simulink model "model_to_linearize"  (R2026a)
settings: Solver=VariableStepAuto
undefined symbols (not defined in the file or in its folder): param
settings Model: Creator=luca  LastModifiedBy=luca

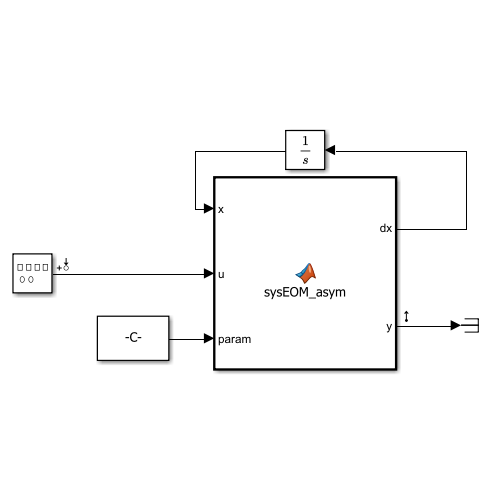
[thumbnail: Simulink's stored preview of the top-level diagram]
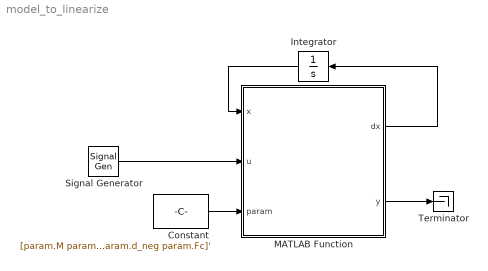
== system model_to_linearize ==
  Constant : Constant  Value=[param.M param.m param.b param.c param.l param.k_pos param.k_neg param.d_pos param.d_neg param.Fc]'
  Integrator : Integrator  InitialCondition=[0; 0; pi; 0]
  MATLAB Function : MATLAB Function  TreatAsAtomicUnit=on
  Signal Generator : SignalGenerator  Units=rad/sec
  Terminator : Terminator
  wires:
  Constant/1 -> MATLAB Function/3(param)
  MATLAB Function/1(dx) -> Integrator/1
  Integrator/1 -> MATLAB Function/1(x)
  MATLAB Function/2(y) -> Terminator/1
  Signal Generator/1 -> MATLAB Function/2(u)

== matlab function model_to_linearize/MATLAB Function ==
  data: x input; u input; dx output; y output; param input
function [dx, y] = sysEOM_asym( x, u,param)
% x = [x, v, \theta, \omega]
% y = [x, \theta]
% Input map: smooth asymmetric gain + asymmetric dead zone
%   F(u) ~ k_pos*(u - d_pos)  for u >  d_pos
%   F(u) ~ k_neg*(u + d_neg)  for u < -d_neg
%   F(u) ~ 0                  otherwise
% Smoothed via sp(z) = 0.5*(z + sqrt(z^2 + eps_sm^2)), a C^inf max(z,0).
% Cart friction: viscous c*v + Coulomb Fc*tanh(eps_c*v) (smooth sign).
M = param(1);
m = param(2);
b = param(3);
c = param(4);
l = param(5);
k_pos = param(6);
k_neg = param(7);
d_pos = param(8);
d_neg = param(9);
Fc = param(10);

g       = 9.81;
eps_sm  = 1e-3; % smoothing width on the input map  (fixed, not estimated)
eps_c   = 30;   % Coulomb tanh sharpness on cart vel (fixed, not estimated)

sp = @(z) 0.5*(z + sqrt(z.^2 + eps_sm^2));
F  = k_pos * sp(u - d_pos) - k_neg * sp(-(u + d_neg));

Delta = M + m*sin(x(3))^2;

num1 = F - c*x(2) - Fc*tanh(eps_c*x(2)) - m*l*x(4)^2*sin(x(3)) ...
       - m*g*cos(x(3))*sin(x(3)) - (b/l)*cos(x(3))*x(4);

num2 = m*l*cos(x(3))*num1 - (M+m)*(m*g*l*sin(x(3)) + b*x(4));

dx = zeros(4,1);
dx(1) = x(2);
dx(2) = num1 / Delta;
dx(3) = x(4);
dx(4) = num2 / (m*l^2 * Delta);

y = [x(1), x(3)]';
end
